simulink model "recepteur_usrp"  (R2020b)
settings: Solver=FixedStepDiscrete  StartTime=0.0  StopTime=0.01  RelTol=1e-3
InitFcn:
  | %%% SELECTIONNEZ LES PARAMETRES DU MODELE %%%
  | 
  | Te = 20e-6;    % temps entre deux échantillons au niveau du canal
  | N = 82;                % nombre total de sous-porteuses
  | pilots_inter = 3;      % nombre de sous-canaux entre deux pilotes
  | prefix_len = 2;      % taille du préfixe cyclique
  | 
  | 
  | %%% NE PAS MODIFIER %%%
  | 
  | pilots_per_sym = 16; % nombre de pilotes par symbole OFDM
  | 
  | N_data = 64;
  | 
  | %TsOFDM = N*Te; % temps symbole OFDM
  | 
  | 
  | %{
  | Te=20e-6;
  | 
  | N=64;
  | 
  | Nb_symboles_trame=10;
  | 
  | pilots_rate=0.25;
  | 
  | Nact=N-1;
  | N_carriers=Nact-N*pilots_rate;
  | 
  | nu=2;  % nombre d'échantillons du préfixe cyclique
  | 
  | Ts=N * Te;
  | Ts_reel=(N+nu)*Te;
  | 
  | L=N/2  % longueur du demi-symbole utile (excluant le préfixe cyclique)
  | 
  | 
  | str='coucou';
  | message=[dec2bin(str,8)=='1'; zeros(11-strlength(str),8)];
  | %}
libraries: dspindex x3, commutil2 x1, dspxfrm3 x1, commdigbbndpm3 x1
Description:
  | This model uses Universal Software Radio Peripheral (USRP) hardware with Simulink(R) to perform FM demodulation and stereo decoding.
settings Model: Creator=nlevrard  LastModifiedBy=nlevrard
settings DataIOCC: SaveFormat=Structure  SaveOutput=off  SignalLogging=off  DSMLogging=off  SaveTime=off  ReturnWorkspaceOutputs=off
settings OptimizationCC: ExpressionDepthLimit=2147483647  EfficientMapNaN2IntZero=off  LifeSpan=inf  SimCompilerOptimization=on
settings DebuggingCC: UnderspecifiedInitializationDetection=Classic  MergeDetectMultiDrivingBlocksExec=none  SolverPrmCheckMsg=warning  InheritedTsInSrcMsg=none  MultiTaskCondExecSysMsg=none  ParameterPrecisionLossMsg=none  FcnCallInpInsideContextMsg=warning  AllowSymbolicDim=off  StateNameClashWarn=warning  SFUnexpectedBacktrackingDiag=warning  SFNoUnconditionalDefaultTransitionDiag=warning  SFExecutionAtInitializationDiag=none  ArithmeticOperatorsInVariantConditions=warning
settings HardwareCC: ProdBitPerPointer=32  ProdBitPerSizeT=32  ProdBitPerPtrDiffT=32  ProdLargestAtomicFloat=None  ProdIntDivRoundTo=Undefined  ProdEndianess=Unspecified  ProdWordSize=32  ProdHWDeviceType=32-bit Generic  TargetBitPerPointer=64  TargetBitPerSizeT=64  TargetBitPerPtrDiffT=64  TargetLongLongMode=on  TargetIntDivRoundTo=Zero  TargetEndianess=LittleEndian  TargetWordSize=64  TargetHWDeviceType=Generic->MATLAB Host Computer  ProdEqTarget=off
settings ModelReferenceCC: PropagateSignalLabelsOutOfModel=off
settings SFSimCC: SimIntegrity=off  SimUseLocalCustomCode=off  CustomCodeUndefinedFunction=UseInterfaceOnly
settings RTWCC: RTWUseLocalCustomCode=off
settings RTWCC: CustomSourceCode=|
  | #include <stdio.h>
  | #include <stdlib.h>
settings CodeAppCC: MaxIdLength=128  StateflowObjectComments=on
settings GRTTargetCC: TargetLangStandard=C89/C90 (ANSI)  CombineOutputUpdateFcns=off  GRTInterface=on
settings ConfigComp: CovMetricSettings=dw  CovSaveCumulativeToWorkspaceVar=on  CovSaveSingleToWorkspaceVar=on  CovExternalEMLEnable=off  CovSFcnEnable=off

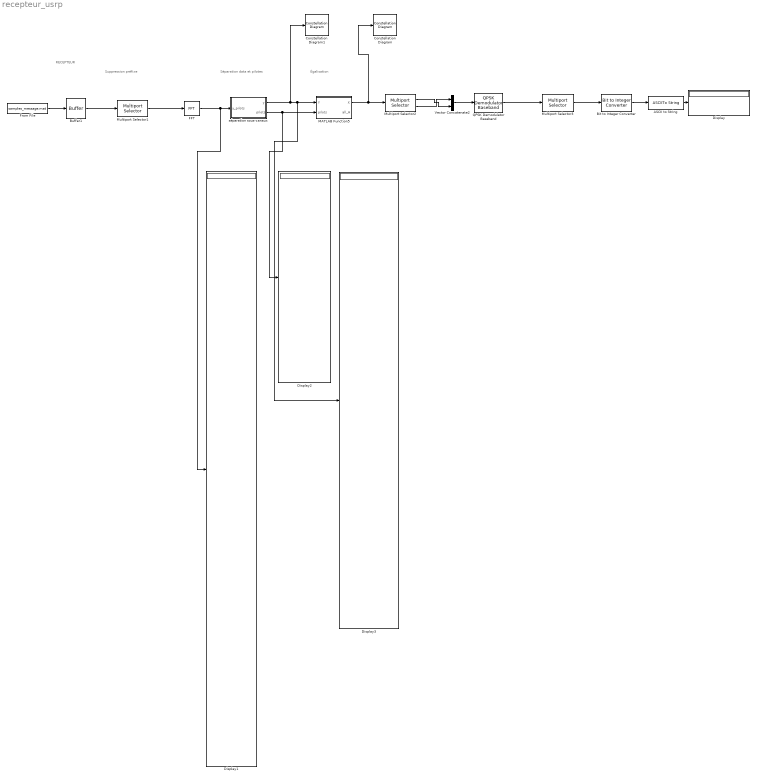
== system recepteur_usrp ==
  note: RECEPTEUR
  note: Égalisation
  note: Séparation data et pilotes
  note: Suppression préfixe
  ASCII to String : ASCIIToString
  Bit to Integer Converter : commutil2/Bit to Integer Converter  nbits=8  bitOrder=MSB first  signedOutputValues=Unsigned  outDtype=uint8  outDtypeSigned=Inherit via internal rule
  Buffer1 : Buffer  N=82  OutputFrames=off
  Constellation Diagram : ConstellationDiagram
  Constellation Diagram1 : ConstellationDiagram
  Display{,1..3} (4 alike) : Display
  FFT : dspxfrm3/FFT  FFTImplementation=Auto  CompMethod=Table lookup  TableOpt=NEW  TableOptActive=Speed  BitRevOrder=off  Normalize=off  InheritFFTLength=on  FFTLength=64  WrapInput=on  roundingMode=Floor  overflowMode=off  firstCoeffDataTypeStr=Inherit: Same word length as input  firstCoeffLastDataTypeStr=Inherit: Same word length as input  outputMin=[]  outputMax=[]
  From File : FromFile  FileName=samples_message.mat  SampleTime=Te  ExtrapolationAfterLastDataPoint=Ground value
  MATLAB Function5 : MATLAB Function  TreatAsAtomicUnit=on
  Multiport Selector1 : dspindex/Multiport Selector  rowsOrCols=Rows  idxCellArray=[ prefix_len + 1 : N]  idxErrMode=Clip Index
  Multiport Selector2 : dspindex/Multiport Selector  rowsOrCols=Rows  idxCellArray={1 : N_data/2, N_data/2+1 : N_data}  idxErrMode=Clip Index
  Multiport Selector3 : dspindex/Multiport Selector  rowsOrCols=Rows  idxCellArray=[ 1 : 88]  idxErrMode=Clip Index
  QPSK Demodulator Baseband : commdigbbndpm3/QPSK Demodulator Baseband  OutType=Bit  DecType=Hard decision  VarSource=Dialog  Variance=1  Dec=Gray  Ph=pi/4  outDtype1=Inherit via internal rule  outDtype2=Inherit via internal rule  derotateFactorWordLen=16  derotateFactorDataTypeStr=Inherit: Same word length as input  derotateFactorLastDataTypeStr=Inherit: Same word length as input
  Vector Concatenate2 : Concatenate
  séparation sous-canaux : MATLAB Function  TreatAsAtomicUnit=on
  wires:
  Bit to Integer Converter/1 -> ASCII to String/1
  ASCII to String/1 -> Display/1
  Multiport Selector2/2 -> Vector Concatenate2/1
  Buffer1/1 -> Multiport Selector1/1
  MATLAB Function5/1(X) -> Constellation Diagram/1, Multiport Selector2/1
  FFT/1 -> Display1/1, séparation sous-canaux/1(y_pilots)
  Multiport Selector1/1 -> FFT/1
  séparation sous-canaux/1(y) -> Constellation Diagram1/1, Display3/1, MATLAB Function5/1(Y)
  séparation sous-canaux/2(pilots) -> Display2/1, MATLAB Function5/2(pilots)
  Multiport Selector2/1 -> Vector Concatenate2/2
  Vector Concatenate2/1 -> QPSK Demodulator Baseband/1
  From File/1 -> Buffer1/1
  Multiport Selector3/1 -> Bit to Integer Converter/1
  QPSK Demodulator Baseband/1 -> Multiport Selector3/1

== matlab function recepteur_usrp/séparation sous-canaux ==
  data: y_pilots input; y output; pilots output; pilots_inter parameter; pilots_per_sym parameter; N_data parameter
function [y, pilots] = fcn(y_pilots, pilots_inter, pilots_per_sym, N_data)

pilots = complex(0, 0) * ones(pilots_per_sym+1, 1);
y = complex(0, 0) * ones(N_data, 1);

pilots(1) = y_pilots(1);

p_counter = 2;
s_counter = 1;

for idx = 2:81
    if mod(idx, pilots_inter+1) ~= 0
        y(s_counter) = y_pilots(idx);
        s_counter = s_counter + 1;
    else
       pilots(p_counter) = y_pilots(idx);
       p_counter = p_counter + 1;
    end
end



%{
pilots = in(1:channels_per_pilot+2:length(in)); % vecteur contenant tous les pilotes du symbole

dup_pilots_bis = complex((1:30), (1:30));
dup_pilots_bis(1) = pilots(1);

for i = 2:length(pilots)-1
    dup_pilots_bis(2*(i-2)+2) = pilots(i);
    dup_pilots_bis(2*(i-2)+2+1) = pilots(i);
end

dup_pilots_bis(end) = pilots(end);

dup_pilots = dup_pilots_bis';


Y = in(setdiff(1:length(i), 1:channels_per_pilot+1:length(i))); % vecteur contenant tous les échantillons du symbole      
%}

== matlab function recepteur_usrp/MATLAB Function5 ==
  data: Y input; X output; pilots input; pilots_per_sym parameter; N_data parameter; pilots_inter parameter; all_H output
function [X,all_H] = fcn(Y, pilots, pilots_per_sym, N_data, pilots_inter)

%ReY = real(Y);
%ImY = imag(Y);

X = complex(0, 0) * ones(N_data, 1);
all_H = complex(0, 0) * ones(N_data, 1); %tmp


right_pilot = pilots(2);
right_H = right_pilot/(1+1i);

X(1) = Y(1)/right_H;
X(2) = Y(2)/right_H;

for bloc_idx = 1:pilots_per_sym-2
    left_pilot = pilots(bloc_idx+1);
    right_pilot = pilots(bloc_idx+2);

    %left_H = complex(real(left_pilot)/10, imag(left_pilot)/10);
    %right_H = complex(real(right_pilot)/10, imag(right_pilot)/10);

    left_H = left_pilot/(1+1i);
    right_H = right_pilot/(1+1i);

    pilots_interp = linspace(left_H, right_H, pilots_inter + 2);

    H_interp = pilots_interp(2:end-1);

    %ReH = real(H_interp);
    %ImH = imag(H_interp);

   for sample = 0:pilots_inter-1
       %ReY_s = ReY(pilots_inter*bloc_idx+sample);
       %ImY_s = ImY(pilots_inter*bloc_idx+sample);
       Y_s = Y(pilots_inter*bloc_idx+sample);

       %X(pilots_inter*bloc_idx+sample) = complex( ReY_s./ReH(sample), ImY_s./ImH(sample) );
       X(pilots_inter*bloc_idx+sample) = Y_s/H_interp(sample);
       %all_H(pilots_inter*bloc_idx+sample) = complex(ReH(sample), ImH(sample));
       all_H(pilots_inter*bloc_idx+sample) = H_interp(sample);
   end

end
